simulink model "House"  (R2022b)
settings: Solver=VariableStepAuto  StartTime=0.0  StopTime=60  RelTol=1e-3
libraries: simulink_extras x1
settings Model: Creator=19860  LastModifiedBy=beikuzi
settings SolverCC: ZeroCrossAlgorithm=Adaptive
settings DebuggingCC: IgnoredZcDiagnostic=none

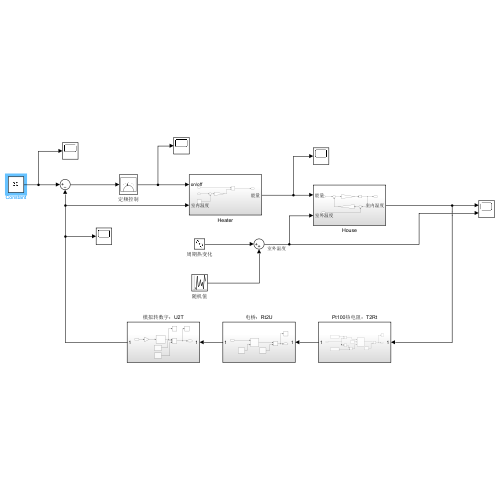
[thumbnail: Simulink's stored preview of the top-level diagram]
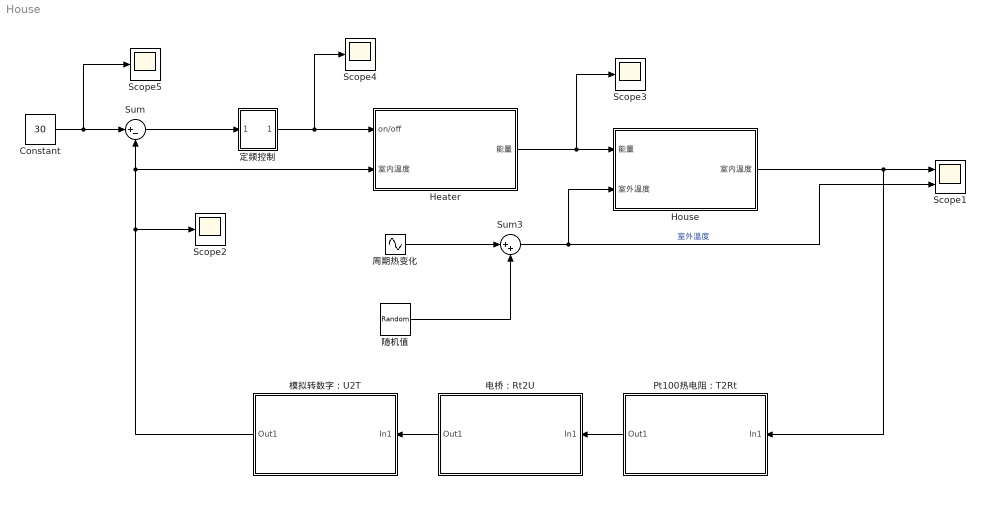
== system House ==
  Constant : Constant  Value=30
  Heater : Subsystem
  House : Subsystem
  Pt100热电阻：T2Rt : Subsystem
  Scope1 : Scope  NumInputPorts=2
  Scope{2..5} (4 alike) : Scope
  Sum : Sum  Inputs=|+-
  Sum3 : Sum  Inputs=|++  InputSameDT=on  SaturateOnIntegerOverflow=on  OutDataTypeStr=Inherit: Same as first input
  周期热变化 : Sin  Amplitude=6  Bias=10  Frequency=2*pi/4  SampleTime=0
  定频控制 : Subsystem
      mask Display: image(fullfile(matlabroot,'toolbox','simulink','simdemos','simgeneral','images','HouseHeatThermostatPix.svg'))
  模拟转数字：U2T : Subsystem
  电桥：Rt2U : Subsystem
  随机值 : UniformRandomNumber  SampleTime=0.1
  wires:
  模拟转数字：U2T/1(Out1) -> Scope2/1, Heater/2(室内温度), Sum/2
  Constant/1 -> Scope5/1, Sum/1
  House/1(室内温度) -> Scope1/1, Pt100热电阻：T2Rt/1(In1)
  Heater/1(能量) -> Scope3/1, House/1(能量)
  Pt100热电阻：T2Rt/1(Out1) -> 电桥：Rt2U/1(In1)
  电桥：Rt2U/1(Out1) -> 模拟转数字：U2T/1(In1)
  定频控制/1(Blower switch) -> Scope4/1, Heater/1(on/off)
  Sum/1 -> 定频控制/1(Terr)
  周期热变化/1 -> Sum3/1
  随机值/1 -> Sum3/2
  Sum3/1 -> Scope1/2, House/2(室外温度)  "室外温度"

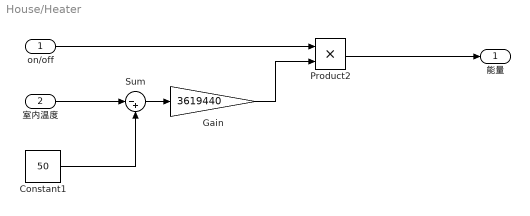
== system House/Heater ==
  on/off : Inport  OutMin=[0]  OutMax=[1]
  室内温度 : Inport  Port=2
  Constant1 : Constant  Value=50
  Gain : Gain  Gain=3619440
  Product2 : Product
  Sum : Sum  Inputs=|-+
  能量 : Outport
  wires:
  室内温度/1 -> Sum/1
  Constant1/1 -> Sum/2
  Sum/1 -> Gain/1
  on/off/1 -> Product2/1
  Gain/1 -> Product2/2
  Product2/1 -> 能量/1

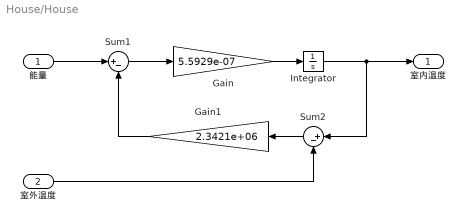
== system House/House ==
  能量 : Inport  OutMin=[0]  OutMax=[1]
  室外温度 : Inport  Port=2
  Gain : Gain  Gain=5.5929e-07
  Gain1 : Gain  Gain=2.3421e+06
  Integrator : Integrator  InitialCondition=20
  Sum1 : Sum  Inputs=|+-
  Sum2 : Sum  Inputs=|+-
  室内温度 : Outport
  wires:
  室外温度/1 -> Sum2/2
  能量/1 -> Sum1/1
  Sum1/1 -> Gain/1
  Sum2/1 -> Gain1/1
  Gain1/1 -> Sum1/2
  Gain/1 -> Integrator/1
  Integrator/1 -> Sum2/1, 室内温度/1

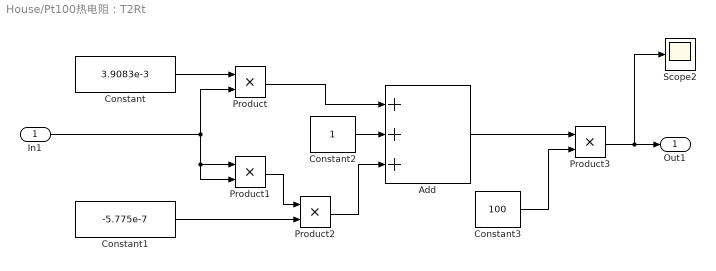
== system House/Pt100热电阻：T2Rt ==
  In1 : Inport
  Add : Sum  Inputs=+++
  Constant : Constant  Value=3.9083e-3
  Constant1 : Constant  Value=-5.775e-7
  Constant2 : Constant
  Constant3 : Constant  Value=100
  Product{,1..3} (4 alike) : Product
  Scope2 : Scope
  Out1 : Outport
  wires:
  In1/1 -> Product/2, Product1/2, Product1/1
  Constant/1 -> Product/1
  Constant1/1 -> Product2/2
  Product1/1 -> Product2/1
  Product/1 -> Add/1
  Product2/1 -> Add/3
  Constant2/1 -> Add/2
  Product3/1 -> Scope2/1, Out1/1
  Add/1 -> Product3/1
  Constant3/1 -> Product3/2

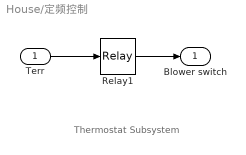
== system House/定频控制 ==
  note: Thermostat Subsystem
  Terr : Inport
  Relay1 : Relay  OnSwitchValue=2  OffSwitchValue=-2
  Blower switch : Outport  InitialOutput=0  VectorParamsAs1DForOutWhenUnconnected=off
  wires:
  Terr/1 -> Relay1/1
  Relay1/1 -> Blower switch/1

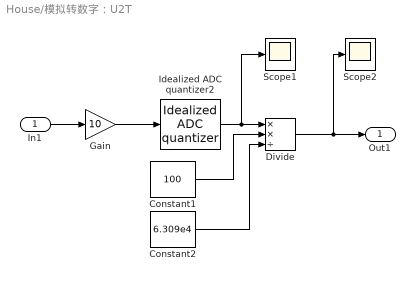
== system House/模拟转数字：U2T ==
  In1 : Inport
  Constant1 : Constant  Value=100
  Constant2 : Constant  Value=6.309e4
  Divide : Product  Inputs=**/
  Gain : Gain  Gain=10
  Idealized ADC quantizer2 : simulink_extras/Additional Discrete/Idealized ADC quantizer  NumberOfConverterBits=16  Vmin=0  Vmax=5  OutputDataType=int32  OutputNegativeValues=off
  Scope1 : Scope
  Scope2 : Scope
  Out1 : Outport
  wires:
  Idealized ADC quantizer2/1 -> Scope1/1, Divide/1
  Constant1/1 -> Divide/2
  Constant2/1 -> Divide/3
  Divide/1 -> Scope2/1, Out1/1
  In1/1 -> Gain/1
  Gain/1 -> Idealized ADC quantizer2/1

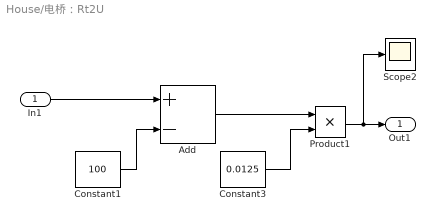
== system House/电桥：Rt2U ==
  In1 : Inport
  Add : Sum  Inputs=+-
  Constant1 : Constant  Value=100
  Constant3 : Constant  Value=0.0125
  Product1 : Product
  Scope2 : Scope
  Out1 : Outport
  wires:
  In1/1 -> Add/1
  Constant1/1 -> Add/2
  Add/1 -> Product1/1
  Constant3/1 -> Product1/2
  Product1/1 -> Scope2/1, Out1/1
